simulink library "INT_RngMod_TrqFrcAdpt"  (R2016b)
settings: Solver=VariableStepAuto  StartTime=0.0  StopTime=10.0  RelTol=1e-3
settings Model: Creator=Administrator  LastModifiedBy=Administrator

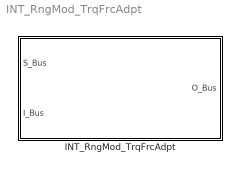
== system INT_RngMod_TrqFrcAdpt ==
  INT_RngMod_TrqFrcAdpt : Subsystem

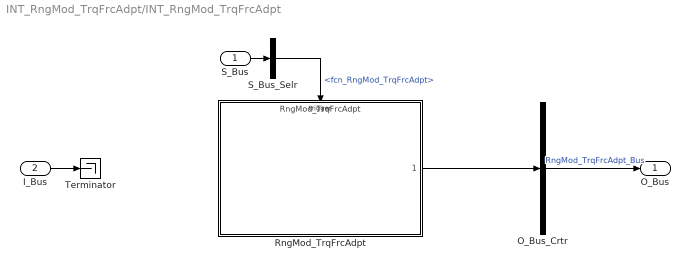
== system INT_RngMod_TrqFrcAdpt/INT_RngMod_TrqFrcAdpt ==
  S_Bus : Inport
  I_Bus : Inport  Port=2
  O_Bus_Crtr : BusCreator  Inputs=1
  RngMod_TrqFrcAdpt : ModelReference  ModelNameDialog=RngMod_TrqFrcAdpt  SimulationMode=Normal  ModelReferenceVersion=1.2  TriggerPortName=function  TriggerPortTriggerType=function-call  TriggerPortStatesWhenEnabling=held
  S_Bus_Selr : BusSelector  OutputSignals=fcn_RngMod_TrqFrcAdpt
  Terminator : Terminator
  O_Bus : Outport
  wires:
  S_Bus_Selr/1 -> RngMod_TrqFrcAdpt/Trigger  "<fcn_RngMod_TrqFrcAdpt>"
  S_Bus/1 -> S_Bus_Selr/1
  I_Bus/1 -> Terminator/1
  O_Bus_Crtr/1 -> O_Bus/1  "RngMod_TrqFrcAdpt_Bus"
  RngMod_TrqFrcAdpt/1 -> O_Bus_Crtr/1
